simulink library "RobotStateLibrary_R2020b"  (R2020b)
settings: Solver=VariableStepAuto  StartTime=0.0  StopTime=10.0  RelTol=1e-3
undefined symbols (not defined in the file or in its folder): Aeq_add, baseFrameName1, basePosePortName, beq_add, config, Config, ConfigRobot1, configSafety, contactFrame1Name, contactFrame2Name, frame1, frame2, frame3, frame4, frameName2, gainStruct, RegStruct, regularization, sampleTime, tollerance, useConstraint, weight
libraries: WBToolboxLibrary x38, $bdroot x32
(part 2 of 2)

== system RobotStateLibrary_R2020b/emergency stop: joint limits/STOP IF THERE ARE SPIKES IN THE ENCODERS ==
  jointPos : Inport
  Enable : EnablePort
  Assertion : Assertion
  MATLAB Function : MATLAB Function  TreatAsAtomicUnit=on
  Unit Delay : UnitDelay  InitialCondition=1  SampleTime=Config.tStep  HasFrameUpgradeWarning=on
  index1 : Constant  Value=Safety.maxJointsPositionDelta  VectorParams1D=off
  check_spikes_joint_pos : Outport
  wires:
  jointPos/1 -> MATLAB Function/1(u)
  MATLAB Function/1(noSpikes) -> Unit Delay/1
  index1/1 -> MATLAB Function/2(delta_u_max)
  MATLAB Function/2(res_check_spikes) -> check_spikes_joint_pos/1
  Unit Delay/1 -> Assertion/1

== matlab function RobotStateLibrary_R2020b/Compute Base Transform from two links/Rotation Average ==
  data: w_H_1 input; w_H output; w_H_2 input
function w_H = rotationAverageFCN(w_H_1, w_H_2)

w_H = rsl.rotationAverage(w_H_1, w_H_2);

end

== matlab function RobotStateLibrary_R2020b/Compute State Velocity/Compute Base Velocity ==
  data: J_contact_1 input; J_contact_2 input; nu_b output; jointVel input; regularization parameter
function nu_b = computeBaseVelocityFCN(J_contact_1, J_contact_2, jointVel, regularization)

    nu_b = rsl.computeBaseVelocityFromContacts(J_contact_1, J_contact_2, jointVel, regularization);

end

== matlab function RobotStateLibrary_R2020b/Force Ergonomy Optimization/Pseudoinverse ==
  data: Aeq input; yMinNorm output; beq input; null output; InvTol parameter
function [yMinNorm, null] = pseudoinverseFCN(Aeq, beq, InvTol)

[yMinNorm, null] = rsl.pseudoinverse(Aeq, beq, InvTol);

end

== matlab function RobotStateLibrary_R2020b/Force Ergonomy Optimization/Prepare QP optimization ==
  data: yMinNorm input; H output; null input; tau_model input; tau_sigma input; Adeq input; bdeq input; g output; A output; ubA output; regularizationHessian parameter; minimizationWeight parameter
function [H, g, A, ubA] = prepareQPOptimizationFCN(yMinNorm, null, tau_model, tau_sigma, Adeq, bdeq, regularizationHessian, minimizationWeight)

[H, g, A, ubA] = rsl.prepareQPOptimization(yMinNorm, null, tau_model, tau_sigma, Adeq, bdeq, regularizationHessian, minimizationWeight);

end

== matlab function RobotStateLibrary_R2020b/State-Machine Reference Generator with Parametrization/State-Machine ==
  data: jointPos input; w_H_base input; jointPos_des output; posCoM input; time input; J input; linkPose input; linkPoseDes input; linkVelocityDes input; phiOld input; posCoM_des output; smoothingTime output; configStateMachine parameter; useSmoothing output; useForwardKinematicsForCoM output; Deltat output; phiOut output; phiNotQP output; H output; f output; Aineq output; bineq output; jointPose_des_old output; jointPose_delta output; useQP output; currentState output
function [jointPos_des, posCoM_des, smoothingTime, useSmoothing, useForwardKinematicsForCoM, Deltat, phiOut, phiNotQP, H, f, Aineq, bineq, jointPose_des_old, jointPose_delta, useQP, currentState] = stateMachineTimeParametrizedFCN(jointPos, w_H_base, posCoM, time, J, linkPose, linkPoseDes, linkVelocityDes, phiOld, configStateMachine)

[jointPos_des, posCoM_des, smoothingTime, useSmoothing, useForwardKinematicsForCoM, Deltat, phiOut, phiNotQP, H, f, Aineq, bineq, jointPose_des_old, jointPose_delta, useQP, currentState] = rsl.stateMachineTimeParametrized(jointPos, w_H_base, posCoM, time, J, linkPose, linkPoseDes, linkVelocityDes, phiOld, configStateMachine);

end

== matlab function RobotStateLibrary_R2020b/emergency stop: joint limits/STOP IF REQUESTED JOINT TORQUES REACH THE LIMITS/MATLAB Function ==
  data: umin input; umax input; u input; inRange output; tol input; res_check_range output
function [inRange, res_check_range] = checkInputRangeFCN(umin, umax, u, tol)

     [inRange, res_check_range] = wbc.checkInputRange(umin, umax, u, tol);
end

== matlab function RobotStateLibrary_R2020b/emergency stop: joint limits/STOP IF THERE ARE SPIKES IN THE ENCODERS/MATLAB Function ==
  data: u input; delta_u_max input; noSpikes output; res_check_spikes output
function [noSpikes, res_check_spikes] = checkInputSpikesFCN(u, delta_u_max)

     [noSpikes, res_check_spikes] = wbc.checkInputSpikes(u, delta_u_max);
end

== matlab function RobotStateLibrary_R2020b/emergency stop: joint limits/STOP IF JOINTS HIT THE LIMITS/MATLAB Function ==
  data: umin input; umax input; u input; inRange output; tol input; res_check_range output
function [inRange, res_check_range] = checkInputRangeFCN(umin, umax, u, tol)

     [inRange, res_check_range] = wbc.checkInputRange(umin, umax, u, tol);
end

== matlab function RobotStateLibrary_R2020b/Postural Task Controller/Postural Task Controller ==
  data: jointPos input; nu input; J input; tau_0_model output; M input; h input; jointPos_des input; jointVel_des input; tau_0_sigma output; GainPostural parameter
function [tau_0_model, tau_0_sigma] =  posturalTaskControllerFCN(jointPos, nu, J, M, h, jointPos_des, jointVel_des, GainPostural)

[tau_0_model, tau_0_sigma] = rsl.posturalTaskController(jointPos, nu, J, M, h, jointPos_des, jointVel_des, GainPostural);

end

== matlab function RobotStateLibrary_R2020b/Pose Yarp Publisher/Transform Matrix to quaternion and position ==
  data: w_H input; q output
function q = transformMatrixToPositionQuaternion_FCN(w_H)

q = wbc.fromTransfMatrixToPosQuat(w_H);

== matlab function RobotStateLibrary_R2020b/Momentum Controller/Momentum Controller Wrench ==
  data: L input; pos_CoM input; desired_pos_vel_acc_CoM input; w_H_meas input; w_R_des input; w_H_contacts input; mass input; wrench_Aeq output; wrench_beq output; wrench_Adeq output; wrench_bdeq output; constraintsMatrixA input; constraintsVectorb input; linksUseConstraintMatrix parameter; GainMomentum parameter
function [wrench_Aeq, wrench_beq, wrench_Adeq, wrench_bdeq] =  momentumControllerWrenchFCN(L, pos_CoM, desired_pos_vel_acc_CoM, w_H_meas, w_R_des, w_H_contacts, mass, constraintsMatrixA, constraintsVectorb, linksUseConstraintMatrix, GainMomentum)

[wrench_Aeq, wrench_beq, wrench_Adeq, wrench_bdeq] = rsl.momentumControllerWrench(L, pos_CoM, desired_pos_vel_acc_CoM, w_H_meas, w_R_des, w_H_contacts, mass, constraintsMatrixA, constraintsVectorb, linksUseConstraintMatrix, GainMomentum);

end

== matlab function RobotStateLibrary_R2020b/Inverse Dynamics/Inverse Dynamics ==
  data: tau_model output; tau_0_model input; tau_0_sigma input; J input; JDot_nu input; M input; h input; B input; tau_sigma output; Reg parameter; fixedLinkVelcityComponents parameter; Lambda output
function [tau_model, tau_sigma, Lambda] = inverseDynamicsFCN(tau_0_model, tau_0_sigma, J, JDot_nu, M, h, B, Reg, fixedLinkVelcityComponents)

[tau_model, tau_sigma, Lambda] = rsl.inverseDynamics(tau_0_model, tau_0_sigma, J, JDot_nu, M, h, B, fixedLinkVelcityComponents, Reg);

end

== matlab function RobotStateLibrary_R2020b/State-Machine Reference Generator/State-Machine ==
  data: jointPos input; jointPos_des output; posCoM input; time input; posCoM_des output; smoothingTime output; configStateMachine parameter; useSmoothing output; useForwardKinematicsForCoM output; currentState output
function [jointPos_des, posCoM_des, smoothingTime, useSmoothing, useForwardKinematicsForCoM, currentState] = stateMachineFCN(jointPos, posCoM, time, configStateMachine)

[jointPos_des, posCoM_des, smoothingTime, useSmoothing, useForwardKinematicsForCoM, currentState] = rsl.stateMachine(jointPos, posCoM, time, configStateMachine);

end
